simulink model "Multistring_inverter"  (R2025a)
settings: Solver=ode1  StartTime=0.0  StopTime=Ttotal  FixedStep=Tsample  MaxStep=1e-3  RelTol=1e-3
values from neighbouring files (symbols this model uses):
  A_0 = 1.5762    [System_parameters.m]
  alpha_T = 0.048/100    (= 0.00048)    [System_parameters.m]
  beta_T = -0.32/100    (= -0.0032)    [System_parameters.m]
  Iscs = Iscs    (= 8.7)    [System_parameters.m]
  Np = 1    [System_parameters.m]
  qk0 = 11594    [System_parameters.m]
  Ttotal = 1e-1    (= 0.1)    [modeling_control_para.m]
  Vocs = Vocs/Ns    (= 0.623333333333)    [System_parameters.m]
settings Model: Creator=mwxiao  LastModifiedBy=yvenk
settings SolverCC: AlgebraicLoopSolver=TrustRegion
settings DataIOCC: LimitDataPoints=on  SaveFormat=Array  SignalLoggingSaveFormat=ModelDataLogs  ReturnWorkspaceOutputs=off  SignalLoggingName=sigsOut
settings OptimizationCC: ExpressionDepthLimit=2147483647.0  LifeSpan=inf
settings DebuggingCC: SaveWithParameterizedLinksMsg=none  UnderspecifiedInitializationDetection=Classic  MergeDetectMultiDrivingBlocksExec=none  SignalResolutionControl=TryResolveAllWithWarning  MultiTaskDSMMsg=warning  MultiTaskCondExecSysMsg=none  FcnCallInpInsideContextMsg=warning  UnconnectedInputMsg=warning  UnconnectedOutputMsg=warning  UnconnectedLineMsg=warning  StateNameClashWarn=warning  SFUnexpectedBacktrackingDiag=warning  SFNoUnconditionalDefaultTransitionDiag=warning  SFExecutionAtInitializationDiag=none  ArithmeticOperatorsInVariantConditions=warning
settings HardwareCC: ProdBitPerPointer=32.0  ProdBitPerSizeT=32.0  ProdBitPerPtrDiffT=32.0  ProdLargestAtomicFloat=None  ProdIntDivRoundTo=Undefined  ProdEndianess=Unspecified  ProdWordSize=32.0  ProdHWDeviceType=32-bit Generic  TargetUnknown=on
settings ModelReferenceCC: PropagateSignalLabelsOutOfModel=off
settings SFSimCC: SimUseLocalCustomCode=off  CustomCodeUndefinedFunction=UseInterfaceOnly
settings RTWCC: RTWUseLocalCustomCode=off  GPUComputeCapability=3.5
settings CodeAppCC: StateflowObjectComments=on
settings GRTTargetCC: TargetLangStandard=C89/C90 (ANSI)  CombineOutputUpdateFcns=off  GRTInterface=on
settings ConfigComp: CovMetricSettings=dw  CovSaveCumulativeToWorkspaceVar=on  CovSaveSingleToWorkspaceVar=on  CovExternalEMLEnable=off

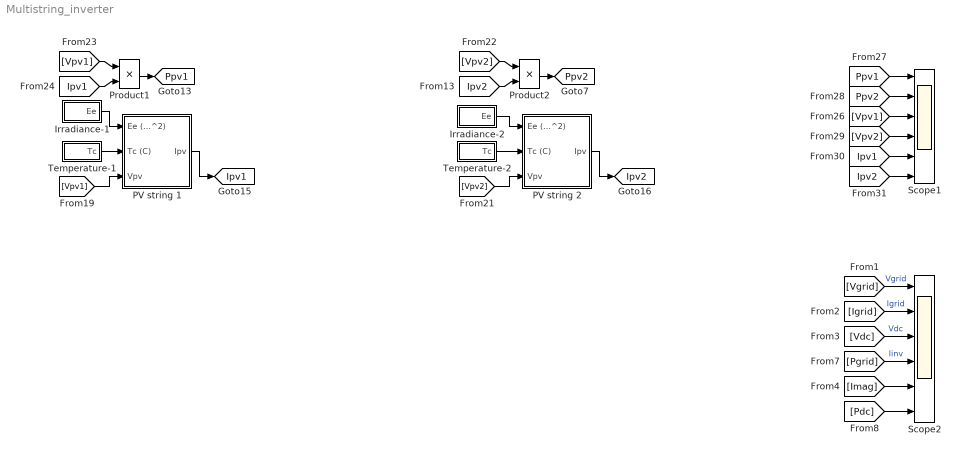
== system Multistring_inverter ==
  Irradiance-1 : Subsystem
  Irradiance-2 : Subsystem
  PV string 1 : Subsystem
      mask Display: image(imread('icon01.jpg'))
  PV string 2 : Subsystem
      mask Display: image(imread('icon01.jpg'))
  Product1 : Product  RndMeth=Zero
  Product2 : Product  RndMeth=Zero
  Scope1 : Scope  NumInputPorts=6
      settings: ActiveDisplayString=5  Title=Ipv1  ShowGrid=off  ActiveDisplayYMinimum=-2.043494935982697  ActiveDisplayYMaximum=7.4160011633406029  DataLoggingVariableName=Simout
  Scope2 : Scope  NumInputPorts=6
      settings: TimeSpan=0.03  ActiveDisplayString=6  Title=Pdc  ActiveDisplayYMinimum=-2110.0991338818271  ActiveDisplayYMaximum=5487.671251020096
  Temperature-1 : Subsystem
  Temperature-2 : Subsystem
  tag scope: Ipv1=global, Ipv2=global, Ppv1=global, Ppv2=global
  wires:
  Irradiance-1/1(Ee) -> PV string 1/1(Ee (W/m^2))
  Temperature-1/1(Tc) -> PV string 1/2(Tc (C))
  [Vpv1] -> PV string 1/3(Vpv)
  PV string 1/1(Ipv) -> [Ipv1]
  Product1/1 -> [Ppv1]
  [Vpv1] -> Product1/1
  [Ipv1] -> Product1/2
  Irradiance-2/1(Ee) -> PV string 2/1(Ee (W/m^2))
  Temperature-2/1(Tc) -> PV string 2/2(Tc (C))
  [Vpv2] -> PV string 2/3(Vpv)
  PV string 2/1(Ipv) -> [Ipv2]
  Product2/1 -> [Ppv2]
  [Vpv2] -> Product2/1
  [Ipv2] -> Product2/2
  [Vgrid] -> Scope2/1  "Vgrid"
  [Igrid] -> Scope2/2  "Igrid"
  [Vdc] -> Scope2/3  "Vdc"
  [Pgrid] -> Scope2/4  "Iinv"
  [Pdc] -> Scope2/6
  [Imag] -> Scope2/5
  [Ppv1] -> Scope1/1
  [Ppv2] -> Scope1/2
  [Vpv1] -> Scope1/3
  [Vpv2] -> Scope1/4
  [Ipv1] -> Scope1/5
  [Ipv2] -> Scope1/6

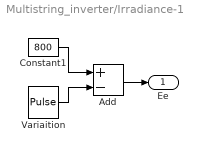
== system Multistring_inverter/Irradiance-1 ==
  Add : Sum  Inputs=+-
  Constant1 : Constant  Value=800
  Variaition : DiscretePulseGenerator  PulseType=Time based  Amplitude=400  Period=Ttotal  PulseWidth=50  PhaseDelay=Ttotal/2+5e-3
  Ee : Outport
  wires:
  Constant1/1 -> Add/1
  Variaition/1 -> Add/2
  Add/1 -> Ee/1

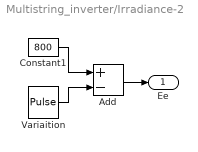
== system Multistring_inverter/Irradiance-2 ==
  Add : Sum  Inputs=+-
  Constant1 : Constant  Value=800
  Variaition : DiscretePulseGenerator  PulseType=Time based  Amplitude=400  Period=Ttotal  PulseWidth=50  PhaseDelay=Ttotal/2+5e-3
  Ee : Outport
  wires:
  Constant1/1 -> Add/1
  Variaition/1 -> Add/2
  Add/1 -> Ee/1

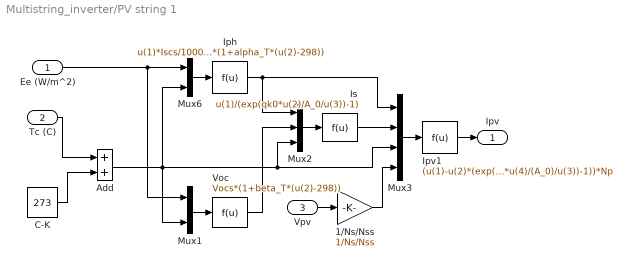
== system Multistring_inverter/PV string 1 ==
  Ee (W/m^2) : Inport
  Tc (C) : Inport  Port=2
  Vpv : Inport  Port=3
  1/Ns/Nss : Gain  Gain=1/Ns/Nss
  Add : Sum
  C-K : Constant  Value=273
  Iph : Fcn  Expr=u(1)*Iscs/1000*(1+alpha_T*(u(2)-298))
  Ipv1 : Fcn  Expr=(u(1)-u(2)*(exp(qk0*u(4)/(A_0)/u(3))-1))*Np
  Is : Fcn  Expr=u(1)/(exp(qk0*u(2)/A_0/u(3))-1)
  Mux1 : Mux  Inputs=2
  Mux2 : Mux  Inputs=3
  Mux3 : Mux
  Mux6 : Mux  Inputs=2
  Voc : Fcn  Expr=Vocs*(1+beta_T*(u(2)-298))
  Ipv : Outport
  wires:
  Mux6/1 -> Iph/1
  Ee (W/m^2)/1 -> Mux6/1, Mux1/1
  Mux1/1 -> Voc/1
  Mux2/1 -> Is/1
  Iph/1 -> Mux2/1, Mux3/1
  Voc/1 -> Mux2/2
  Mux3/1 -> Ipv1/1
  Is/1 -> Mux3/2
  Vpv/1 -> 1/Ns/Nss/1
  Ipv1/1 -> Ipv/1
  Tc (C)/1 -> Add/1
  Add/1 -> Mux6/2, Mux1/2, Mux3/3, Mux2/3
  C-K/1 -> Add/2
  1/Ns/Nss/1 -> Mux3/4

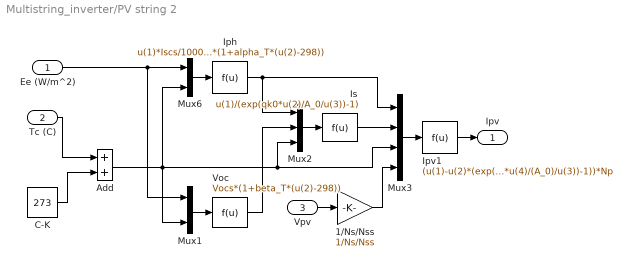
== system Multistring_inverter/PV string 2 ==
  Ee (W/m^2) : Inport
  Tc (C) : Inport  Port=2
  Vpv : Inport  Port=3
  1/Ns/Nss : Gain  Gain=1/Ns/Nss
  Add : Sum
  C-K : Constant  Value=273
  Iph : Fcn  Expr=u(1)*Iscs/1000*(1+alpha_T*(u(2)-298))
  Ipv1 : Fcn  Expr=(u(1)-u(2)*(exp(qk0*u(4)/(A_0)/u(3))-1))*Np
  Is : Fcn  Expr=u(1)/(exp(qk0*u(2)/A_0/u(3))-1)
  Mux1 : Mux  Inputs=2
  Mux2 : Mux  Inputs=3
  Mux3 : Mux
  Mux6 : Mux  Inputs=2
  Voc : Fcn  Expr=Vocs*(1+beta_T*(u(2)-298))
  Ipv : Outport
  wires:
  Mux6/1 -> Iph/1
  Ee (W/m^2)/1 -> Mux6/1, Mux1/1
  Mux1/1 -> Voc/1
  Mux2/1 -> Is/1
  Iph/1 -> Mux2/1, Mux3/1
  Voc/1 -> Mux2/2
  Mux3/1 -> Ipv1/1
  Is/1 -> Mux3/2
  Vpv/1 -> 1/Ns/Nss/1
  Ipv1/1 -> Ipv/1
  Tc (C)/1 -> Add/1
  Add/1 -> Mux6/2, Mux1/2, Mux3/3, Mux2/3
  C-K/1 -> Add/2
  1/Ns/Nss/1 -> Mux3/4

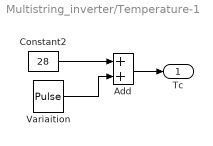
== system Multistring_inverter/Temperature-1 ==
  Add : Sum
  Constant2 : Constant  Value=28
  Variaition : DiscretePulseGenerator  PulseType=Time based  Amplitude=0  Period=20e-3  PulseWidth=50  PhaseDelay=Ttotal/4
  Tc : Outport
  wires:
  Constant2/1 -> Add/1
  Variaition/1 -> Add/2
  Add/1 -> Tc/1

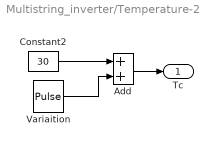
== system Multistring_inverter/Temperature-2 ==
  Add : Sum
  Constant2 : Constant  Value=30
  Variaition : DiscretePulseGenerator  PulseType=Time based  Amplitude=0  Period=20e-3  PulseWidth=50  PhaseDelay=Ttotal/4
  Tc : Outport
  wires:
  Constant2/1 -> Add/1
  Variaition/1 -> Add/2
  Add/1 -> Tc/1
